simulink model "PID_Controller"  (R2018b)
settings: Solver=VariableStepAuto  StartTime=0.0  StopTime=10.0  RelTol=1e-3  EnableMultiTasking=on
values from neighbouring files (symbols this model uses):
  Fmatrix = [-1/sqrt(2) 0 1/sqrt(2) 1 ... (first row only)    [I_F_matrices.m]
  Imatrix = [1 0 0 1/2 ... (first row only)    [I_F_matrices.m]
libraries: simulink_extras x4, dspinverses x1
(part 1 of 3)
settings Model: Creator=as01398  LastModifiedBy=rache
settings DataIOCC: OutputOption=SpecifiedOutputTimes  OutputTimes=[0:0.2:10]
settings OptimizationCC: LifeSpan=inf
settings DebuggingCC: SFUnexpectedBacktrackingDiag=warning  SFNoUnconditionalDefaultTransitionDiag=warning  UnderSpecifiedDimensionMsg=warning
settings SFSimCC: SimUseLocalCustomCode=off
settings RTWCC: RTWUseLocalCustomCode=off
settings CodeAppCC: StateflowObjectComments=on
settings GRTTargetCC: TargetLangStandard=C89/C90 (ANSI)  GeneratePreprocessorConditionals=Disable all
settings ConfigComp: CovMetricSettings=dw  CovHtmlReporting=on  CovSaveCumulativeToWorkspaceVar=on  CovSaveSingleToWorkspaceVar=on  CovExternalEMLEnable=off

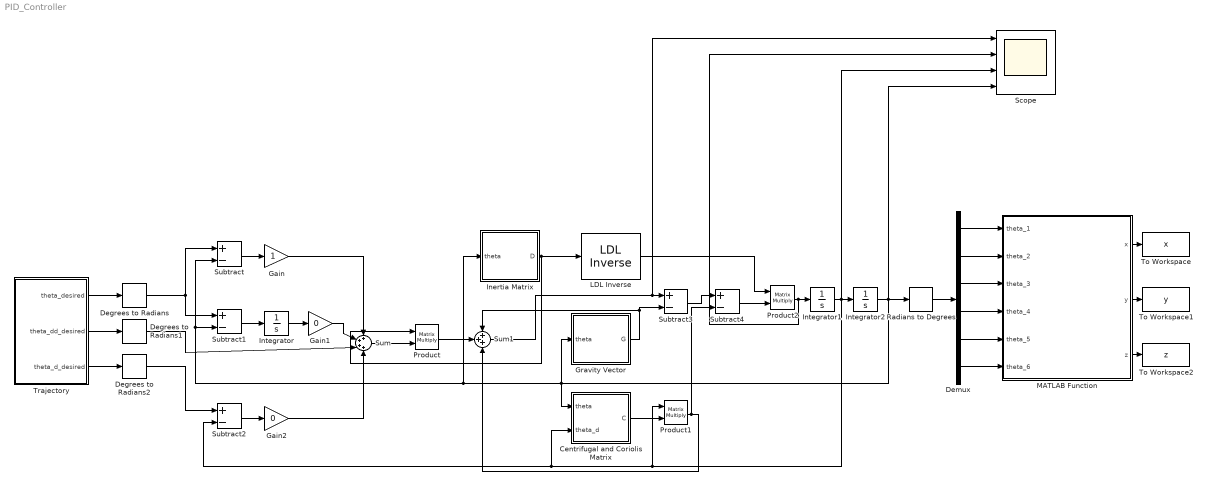
== system PID_Controller ==
  Centrifugal and Coriolis Matrix : Subsystem
  Degrees to Radians : simulink_extras/Transformations/Degrees to Radians
  Degrees to Radians1 : simulink_extras/Transformations/Degrees to Radians
  Degrees to Radians2 : simulink_extras/Transformations/Degrees to Radians
  Demux : Demux  Outputs=6
  Gain : Gain
  Gain1 : Gain  Gain=0
  Gain2 : Gain  Gain=0
  Gravity Vector : Subsystem
  Inertia Matrix : Subsystem
  Integrator : Integrator
  Integrator1 : Integrator
  Integrator2 : Integrator
  LDL Inverse : dspinverses/LDL Inverse  errmode=Warning
      settings: SourceProductName=DSP System Toolbox  SourceProductBaseCode=DS
  MATLAB Function : MATLAB Function  TreatAsAtomicUnit=on
  Product : Product  Multiplication=Matrix(*)
  Product1 : Product  Multiplication=Matrix(*)
  Product2 : Product  Multiplication=Matrix(*)
  Radians to Degrees : simulink_extras/Transformations/Radians to Degrees
  Scope : Scope  NumInputPorts=4
  Subtract{,1..4} (5 alike) : Sum  Inputs=+-
  Sum : Sum  Inputs=4
  Sum1 : Sum  Inputs=3
  To Workspace : ToWorkspace  VariableName=x  SaveFormat=Timeseries  SampleTime=-1
  To Workspace1 : ToWorkspace  VariableName=y  SaveFormat=Timeseries  SampleTime=-1
  To Workspace2 : ToWorkspace  VariableName=z  SaveFormat=Timeseries  SampleTime=-1
  Trajectory : Subsystem
  wires:
  Trajectory/1(theta_desired) -> Degrees to Radians/1
  Trajectory/3(theta_d_desired) -> Degrees to Radians2/1
  Subtract1/1 -> Integrator/1
  Subtract/1 -> Gain/1
  Integrator/1 -> Gain1/1
  Gain1/1 -> Sum/2
  Subtract2/1 -> Gain2/1
  Gain2/1 -> Sum/4
  Gain/1 -> Sum/1
  Trajectory/2(theta_dd_desired) -> Degrees to Radians1/1
  Sum/1 -> Product/2
  Product/1 -> Sum1/2
  Gravity Vector/1(G) -> Subtract3/2, Sum1/1
  Centrifugal and Coriolis Matrix/1(C) -> Product1/2
  Product1/1 -> Subtract4/2, Sum1/3
  Sum1/1 -> Scope/1, Subtract3/1
  Inertia Matrix/1(D) -> LDL Inverse/1, Product/1
  Subtract4/1 -> Product2/2
  Product2/1 -> Scope/2, Integrator1/1
  Integrator1/1 -> Product1/1, Centrifugal and Coriolis Matrix/2(theta_d), Subtract2/2, Scope/3, Integrator2/1
  Integrator2/1 -> Inertia Matrix/1(theta), Subtract1/2, Subtract/2, Centrifugal and Coriolis Matrix/1(theta), Gravity Vector/1(theta), Radians to Degrees/1, Scope/4
  Demux/1 -> MATLAB Function/1(theta_1)
  Demux/2 -> MATLAB Function/2(theta_2)
  Demux/3 -> MATLAB Function/3(theta_3)
  Demux/4 -> MATLAB Function/4(theta_4)
  Demux/5 -> MATLAB Function/5(theta_5)
  Demux/6 -> MATLAB Function/6(theta_6)
  MATLAB Function/1(x) -> To Workspace/1
  MATLAB Function/2(y) -> To Workspace1/1
  MATLAB Function/3(z) -> To Workspace2/1
  Subtract3/1 -> Subtract4/1
  LDL Inverse/1 -> Product2/1
  Degrees to Radians/1 -> Subtract1/1, Subtract/1
  Degrees to Radians1/1 -> Sum/3
  Degrees to Radians2/1 -> Subtract2/1
  Radians to Degrees/1 -> Demux/1

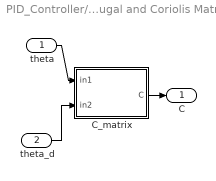
== system PID_Controller/Centrifugal and Coriolis Matrix ==
  theta : Inport
  theta_d : Inport  Port=2
  C_matrix : MATLAB Function  TreatAsAtomicUnit=on
  C : Outport
  wires:
  theta_d/1 -> C_matrix/2(in2)
  theta/1 -> C_matrix/1(in1)
  C_matrix/1(C) -> C/1

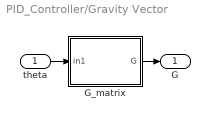
== system PID_Controller/Gravity Vector ==
  theta : Inport
  G_matrix : MATLAB Function  TreatAsAtomicUnit=on
  G : Outport
  wires:
  G_matrix/1(G) -> G/1
  theta/1 -> G_matrix/1(in1)

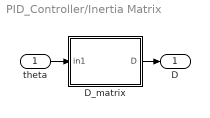
== system PID_Controller/Inertia Matrix ==
  theta : Inport
  D_matrix : MATLAB Function  TreatAsAtomicUnit=on
  D : Outport
  wires:
  D_matrix/1(D) -> D/1
  theta/1 -> D_matrix/1(in1)

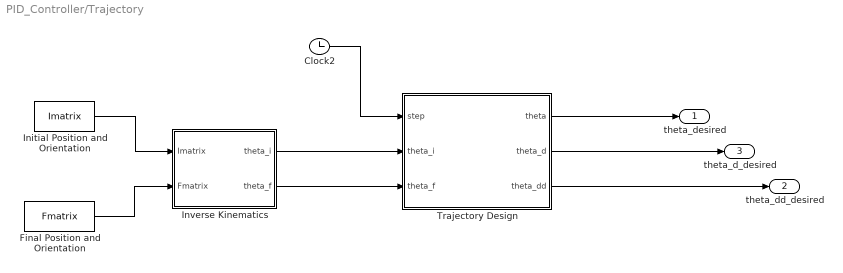
== system PID_Controller/Trajectory ==
  Clock2 : Clock
      settings: Decimation=1000
  Final Position and Orientation : Constant  Value=Fmatrix
  Initial Position and Orientation : Constant  Value=Imatrix
  Inverse Kinematics : MATLAB Function  TreatAsAtomicUnit=on
  Trajectory Design : MATLAB Function  TreatAsAtomicUnit=on
  theta_desired : Outport
  theta_dd_desired : Outport  Port=2
  theta_d_desired : Outport  Port=3
  wires:
  Trajectory Design/3(theta_dd) -> theta_dd_desired/1
  Trajectory Design/2(theta_d) -> theta_d_desired/1
  Trajectory Design/1(theta) -> theta_desired/1
  Inverse Kinematics/2(theta_f) -> Trajectory Design/3(theta_f)
  Inverse Kinematics/1(theta_i) -> Trajectory Design/2(theta_i)
  Final Position and Orientation/1 -> Inverse Kinematics/2(Fmatrix)
  Initial Position and Orientation/1 -> Inverse Kinematics/1(Imatrix)
  Clock2/1 -> Trajectory Design/1(step)
